simulink model "AmplitudeModulation"  (R2023b)
settings: Solver=VariableStepAuto  StartTime=0.0  StopTime=10.0  RelTol=1e-3

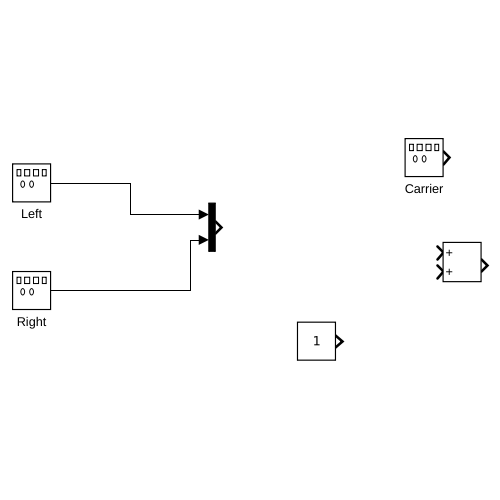
[thumbnail: Simulink's stored preview of the top-level diagram]
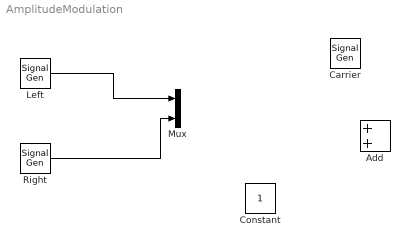
== system AmplitudeModulation ==
  Add : Sum
  Carrier : SignalGenerator  Units=rad/sec
  Constant : Constant
  Left : SignalGenerator  Units=rad/sec
  Mux : Mux  Inputs=2
  Right : SignalGenerator  Units=rad/sec
  wires:
  Left/1 -> Mux/1
  Right/1 -> Mux/2
